simulink model "AMCLIB_FWSpeedLoop_BAM"  (Simulink 9.3)
settings: Solver=VariableStepAuto  StartTime=0.0  StopTime=10.0  RelTol=1e-3
(part 2 of 2)

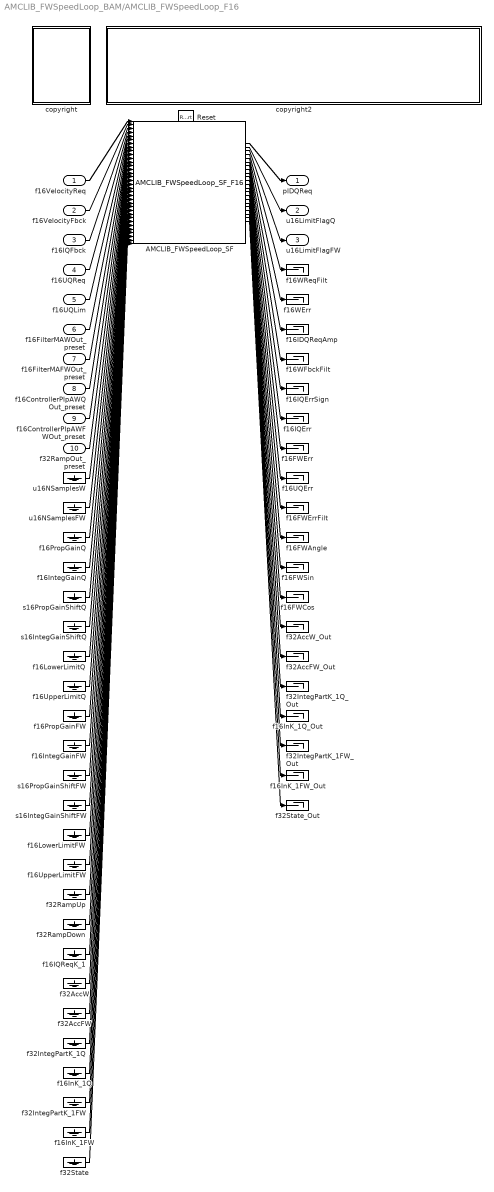
== system AMCLIB_FWSpeedLoop_BAM/AMCLIB_FWSpeedLoop_F16 ==
  f16VelocityReq : Inport  OutDataTypeStr=int16
  f16VelocityFbck : Inport  Port=2  OutDataTypeStr=int16
  f16IQFbck : Inport  Port=3  OutDataTypeStr=int16
  f16UQReq : Inport  Port=4  OutDataTypeStr=int16
  f16UQLim : Inport  Port=5  OutDataTypeStr=int16
  f16FilterMAWOut_preset : Inport  Port=6  OutDataTypeStr=int16
  f16FilterMAFWOut_preset : Inport  Port=7  OutDataTypeStr=int16
  f16ControllerPIpAWQOut_preset : Inport  Port=8  OutDataTypeStr=int16
  f16ControllerPIpAWFWOut_preset : Inport  Port=9  OutDataTypeStr=int16
  f32RampOut_preset : Inport  Port=10  OutDataTypeStr=int32
  Reset : ResetPort  DisableCoverage=on
  AMCLIB_FWSpeedLoop_SF : S-Function  FunctionName=AMCLIB_FWSpeedLoop_SF_F16  Parameters=showStates,resetStatesEnable,showDebugOutputs,u16NSamplesW,u16NSamplesFW,f16PropGainQ,f16IntegGainQ,s16PropGainShiftQ,s16IntegGainShiftQ,f16LowerLimitQ,f16UpperLimitQ,f16PropGainFW,f16IntegGainFW,s16PropGainShiftFW,s16IntegGainShiftFW,f16LowerLimitFW,f16UpperLimitFW,f32RampUp,f32RampDown  SFunctionDeploymentMode=off  EnableBusSupport=off
  copyright : Subsystem
      mask Display: text(10,90,'FILE:');text(10,75,'DESRIPTION:');text(10,60,'COPYRIGHT:');text(10,45,'VERSION:');text(10,30,'DATE:')
  copyright2 : Subsystem
      mask Display: text(10,90,'AMCLIB_FWSpeedLoop_BAM_F16.mdl');text(10,75,'PMSM Speed Loop with Field Weakening.');text(10,60,'NXP 2020');text(10,45,'1.0');text(10,30,'28-Mar-2020');
  f16FWAngle : Terminator
  f16FWCos : Terminator
  f16FWErr : Terminator
  f16FWErrFilt : Terminator
  f16FWSin : Terminator
  f16IDQReqAmp : Terminator
  f16IQErr : Terminator
  f16IQErrSign : Terminator
  f16IQReqK_1 : Ground
  f16InK_1FW : Ground
  f16InK_1FW_Out : Terminator
  f16InK_1Q : Ground
  f16InK_1Q_Out : Terminator
  f16IntegGainFW : Ground
  f16IntegGainQ : Ground
  f16LowerLimitFW : Ground
  f16LowerLimitQ : Ground
  f16PropGainFW : Ground
  f16PropGainQ : Ground
  f16UQErr : Terminator
  f16UpperLimitFW : Ground
  f16UpperLimitQ : Ground
  f16WErr : Terminator
  f16WFbckFilt : Terminator
  f16WReqFilt : Terminator
  f32AccFW : Ground
  f32AccFW_Out : Terminator
  f32AccW : Ground
  f32AccW_Out : Terminator
  f32IntegPartK_1FW : Ground
  f32IntegPartK_1FW_Out : Terminator
  f32IntegPartK_1Q : Ground
  f32IntegPartK_1Q_Out : Terminator
  f32RampDown : Ground
  f32RampUp : Ground
  f32State : Ground
  f32State_Out : Terminator
  s16IntegGainShiftFW : Ground
  s16IntegGainShiftQ : Ground
  s16PropGainShiftFW : Ground
  s16PropGainShiftQ : Ground
  u16NSamplesFW : Ground
  u16NSamplesW : Ground
  pIDQReq : Outport
  u16LimitFlagQ : Outport  Port=2
  u16LimitFlagFW : Outport  Port=3
  wires:
  f16VelocityReq/1 -> AMCLIB_FWSpeedLoop_SF/1
  f16VelocityFbck/1 -> AMCLIB_FWSpeedLoop_SF/2
  f16IQFbck/1 -> AMCLIB_FWSpeedLoop_SF/3
  f16UQReq/1 -> AMCLIB_FWSpeedLoop_SF/4
  f16UQLim/1 -> AMCLIB_FWSpeedLoop_SF/5
  f16FilterMAWOut_preset/1 -> AMCLIB_FWSpeedLoop_SF/6
  f16FilterMAFWOut_preset/1 -> AMCLIB_FWSpeedLoop_SF/7
  f16ControllerPIpAWQOut_preset/1 -> AMCLIB_FWSpeedLoop_SF/8
  f16ControllerPIpAWFWOut_preset/1 -> AMCLIB_FWSpeedLoop_SF/9
  f32RampOut_preset/1 -> AMCLIB_FWSpeedLoop_SF/10
  u16NSamplesW/1 -> AMCLIB_FWSpeedLoop_SF/11
  u16NSamplesFW/1 -> AMCLIB_FWSpeedLoop_SF/12
  f16PropGainQ/1 -> AMCLIB_FWSpeedLoop_SF/13
  f16IntegGainQ/1 -> AMCLIB_FWSpeedLoop_SF/14
  s16PropGainShiftQ/1 -> AMCLIB_FWSpeedLoop_SF/15
  s16IntegGainShiftQ/1 -> AMCLIB_FWSpeedLoop_SF/16
  f16LowerLimitQ/1 -> AMCLIB_FWSpeedLoop_SF/17
  f16UpperLimitQ/1 -> AMCLIB_FWSpeedLoop_SF/18
  f16PropGainFW/1 -> AMCLIB_FWSpeedLoop_SF/19
  f16IntegGainFW/1 -> AMCLIB_FWSpeedLoop_SF/20
  s16PropGainShiftFW/1 -> AMCLIB_FWSpeedLoop_SF/21
  s16IntegGainShiftFW/1 -> AMCLIB_FWSpeedLoop_SF/22
  f16LowerLimitFW/1 -> AMCLIB_FWSpeedLoop_SF/23
  f16UpperLimitFW/1 -> AMCLIB_FWSpeedLoop_SF/24
  f32RampUp/1 -> AMCLIB_FWSpeedLoop_SF/25
  f32RampDown/1 -> AMCLIB_FWSpeedLoop_SF/26
  f16IQReqK_1/1 -> AMCLIB_FWSpeedLoop_SF/27
  f32AccW/1 -> AMCLIB_FWSpeedLoop_SF/28
  f32AccFW/1 -> AMCLIB_FWSpeedLoop_SF/29
  f32IntegPartK_1Q/1 -> AMCLIB_FWSpeedLoop_SF/30
  f16InK_1Q/1 -> AMCLIB_FWSpeedLoop_SF/31
  f32IntegPartK_1FW/1 -> AMCLIB_FWSpeedLoop_SF/32
  f16InK_1FW/1 -> AMCLIB_FWSpeedLoop_SF/33
  f32State/1 -> AMCLIB_FWSpeedLoop_SF/34
  AMCLIB_FWSpeedLoop_SF/1 -> pIDQReq/1
  AMCLIB_FWSpeedLoop_SF/2 -> u16LimitFlagQ/1
  AMCLIB_FWSpeedLoop_SF/3 -> u16LimitFlagFW/1
  AMCLIB_FWSpeedLoop_SF/4 -> f16WReqFilt/1
  AMCLIB_FWSpeedLoop_SF/5 -> f16WErr/1
  AMCLIB_FWSpeedLoop_SF/6 -> f16IDQReqAmp/1
  AMCLIB_FWSpeedLoop_SF/7 -> f16WFbckFilt/1
  AMCLIB_FWSpeedLoop_SF/8 -> f16IQErrSign/1
  AMCLIB_FWSpeedLoop_SF/9 -> f16IQErr/1
  AMCLIB_FWSpeedLoop_SF/10 -> f16FWErr/1
  AMCLIB_FWSpeedLoop_SF/11 -> f16UQErr/1
  AMCLIB_FWSpeedLoop_SF/12 -> f16FWErrFilt/1
  AMCLIB_FWSpeedLoop_SF/13 -> f16FWAngle/1
  AMCLIB_FWSpeedLoop_SF/14 -> f16FWSin/1
  AMCLIB_FWSpeedLoop_SF/15 -> f16FWCos/1
  AMCLIB_FWSpeedLoop_SF/16 -> f32AccW_Out/1
  AMCLIB_FWSpeedLoop_SF/17 -> f32AccFW_Out/1
  AMCLIB_FWSpeedLoop_SF/18 -> f32IntegPartK_1Q_Out/1
  AMCLIB_FWSpeedLoop_SF/19 -> f16InK_1Q_Out/1
  AMCLIB_FWSpeedLoop_SF/20 -> f32IntegPartK_1FW_Out/1
  AMCLIB_FWSpeedLoop_SF/21 -> f16InK_1FW_Out/1
  AMCLIB_FWSpeedLoop_SF/22 -> f32State_Out/1

== system AMCLIB_FWSpeedLoop_BAM/AMCLIB_FWSpeedLoop_F16/copyright ==

== system AMCLIB_FWSpeedLoop_BAM/AMCLIB_FWSpeedLoop_F16/copyright2 ==
